simulink model "SimpleAdaptiveControl"  (R2017b)
settings: Solver=ode4  StartTime=0.0  StopTime=tsim  FixedStep=baseRate  RelTol=1e-3  EnableMultiTasking=on
values from neighbouring files (symbols this model uses):
  alpha = 1    [Run_Initializer.m]
  Cmout = [alpha*eye(3,3),eye(3,3)]    [Run_Initializer.m]
  drop_states_BLACK = [1.79313305664063,1.22521911621094,0.176047682762146]    [Run_Initializer.m]
  drop_states_RED = [2.60644311523438,1.21791186523438,3.08142089843750]    [Run_Initializer.m]
  GeI = 2e-2*eye(3,3)    [Run_Initializer.m]
  GeP = 1e-0*eye(3,3)    [Run_Initializer.m]
  GuI = 1e-2*eye(3,3)    [Run_Initializer.m]
  GuP = 8e-0*eye(3,3)    [Run_Initializer.m]
  GxI = 1e-2*eye(6,6)    [Run_Initializer.m]
  GxP = 8e-0*eye(6,6)    [Run_Initializer.m]
  home_states_BLACK = [ xLength/2; yLength/2; 0]    [Run_Initializer.m]
  home_states_RED = [ xLength/2+0.7; yLength/2; pi]    [Run_Initializer.m]
  init_states_BLACK = [ xLength/2; yLength/2; 0]    [Run_Initializer.m]
  init_states_RED = [ xLength/2+0.7; yLength/2; pi]    [Run_Initializer.m]
  Kd_tb = 0.4    [Run_Initializer.m]
  Kd_tr = 0.4    [Run_Initializer.m]
  Kd_xb = 5    [Run_Initializer.m]
  Kd_xr = 5    [Run_Initializer.m]
  Kd_yb = 5    [Run_Initializer.m]
  Kd_yr = 5    [Run_Initializer.m]
  KeI0 = (1e-4).*[   0.1063   -0.0058         0 ... (first row only)    [Run_Initializer.m]
  Kp_tb = 0.1    [Run_Initializer.m]
  Kp_tr = 0.1    [Run_Initializer.m]
  Kp_xb = 2    [Run_Initializer.m]
  Kp_xr = 2    [Run_Initializer.m]
  Kp_yb = 2    [Run_Initializer.m]
  Kp_yr = 2    [Run_Initializer.m]
  KuI0 = [  -0.0066   -0.0031         0 ... (first row only)    [Run_Initializer.m]
  KxI0 = [  -0.0060   -0.0020         0   -0.0001   -0.0001     0 ... (first row only)    [Run_Initializer.m]
  noise_variance_BLACK = 0    [Run_Initializer.m]
  noise_variance_RED = 0    [Run_Initializer.m]
  Phase0_End = Phase0_Duration    (= 10)    [Run_Initializer.m]
  Phase1_End = Phase0_Duration + Phase1_Duration    (= 15)    [Run_Initializer.m]
  Phase2_End = Phase0_Duration + Phase1_Duration +                                   Phase2_Duration    (= 35)    [Run_Initializer.m]
  Phase3_End = Phase0_Duration + Phase1_Duration +                                   Phase2_Duration + Phase3_Duration    (= 166)    [Run_Initializer.m]
  Phase3_SubPhase1_End = Phase2_End + Phase3_SubPhase1_Duration    (= 40)    [Run_Initializer.m]
  Phase3_SubPhase2_End = Phase2_End + Phase3_SubPhase1_Duration +                                   Phase3_SubPhase2_Duration    (= 45)    [Run_Initializer.m]
  Phase3_SubPhase3_End = Phase2_End + Phase3_SubPhase1_Duration +                                   Phase3_SubPhase2_Duration +                                  Phase3_SubPhase3_Duration    (= 46)    [Run_Initializer.m]
  Phase3_SubPhase4_End = Phase2_End + Phase3_SubPhase1_Duration +                                   Phase3_SubPhase2_Duration +                                  Phase3_SubPhase3_Duration +                                  Phase3_SubPhase4_Duration    [Run_Initializer.m]
  Phase4_End = Phase0_Duration + Phase1_Duration +                                   Phase2_Duration + Phase3_Duration +                                   Phase4_Duration    (= 186)    [Run_Initializer.m]
  Phase5_End = Phase0_Duration + Phase1_Duration +                                   Phase2_Duration + Phase3_Duration +                                   Phase4_Duration + Phase5_Duration    (= 191)    [Run_Initializer.m]
  serverRate = 0.1    [Run_Initializer.m]
  sigma_eI = 0.4    [Run_Initializer.m]
  sigma_uI = 0.4    [Run_Initializer.m]
  sigma_xI = 0.4    [Run_Initializer.m]
  sysd1 = c2d(sys,serverRate,opt)    [Run_Initializer.m]
  xLength = 3.51155    [Run_Initializer.m]
  xm_ini = [xLength/2+0.7, yLength/2, 0, 0, 0, 0]'    [Run_Initializer.m]
  yLength = 2.41935    [Run_Initializer.m]
undefined symbols (not defined in the file or in its folder): DiscIntNeverNeededParam, F_thrusters_BLACK, F_thrusters_RED, platformSelection, simMode, thruster_dist2CG_BLACK, thruster_dist2CG_RED
libraries: MainLibrary x22, GPIOLibrary x20, raspberrypilib x17, embdlinuxlib x6, dspsigops x5, dspswit3 x2
(part 1 of 5)
settings Model: Creator=AlexC  LastModifiedBy=SRCL
settings SolverCC: PositivePriorityOrder=on
settings OptimizationCC: UseFloatMulNetSlope=on  PassReuseOutputArgsThreshold=0  EfficientFloat2IntCast=on  MaxStackSize=64  SimCompilerOptimization=on
settings DebuggingCC: MultiTaskDSMMsg=none  ParameterTunabilityLossMsg=error
settings HardwareCC: ProdBitPerPointer=32  ProdBitPerSizeT=32  ProdBitPerPtrDiffT=32  ProdLargestAtomicInteger=Long  ProdLargestAtomicFloat=Double  ProdWordSize=32  ProdHWDeviceType=ARM Compatible->ARM Cortex
settings SFSimCC: MATLABDynamicMemAlloc=off
settings RTWCC: SystemTargetFile=ert.tlc  HardwareBoard=Raspberry Pi  TemplateMakefile=ert_default_tmf  Toolchain=GNU GCC Raspberry Pi  BuildConfiguration=Faster Runs  TargetLang=C++
settings CodeAppCC: ForceParamTrailComments=on  OperatorAnnotations=on
settings ERTTargetCC: TargetLangStandard=C++03 (ISO)  CombineSignalStateStructs=on  ERTCustomFileBanners=off  MatFileLogging=on  SupportContinuousTime=on  SupportNonInlinedSFcns=on  RemoveResetFunc=off  SupportVariableSizeSignals=on  ModelStepFunctionPrototypeControlCompliant=off  RootIOFormat=Structure reference

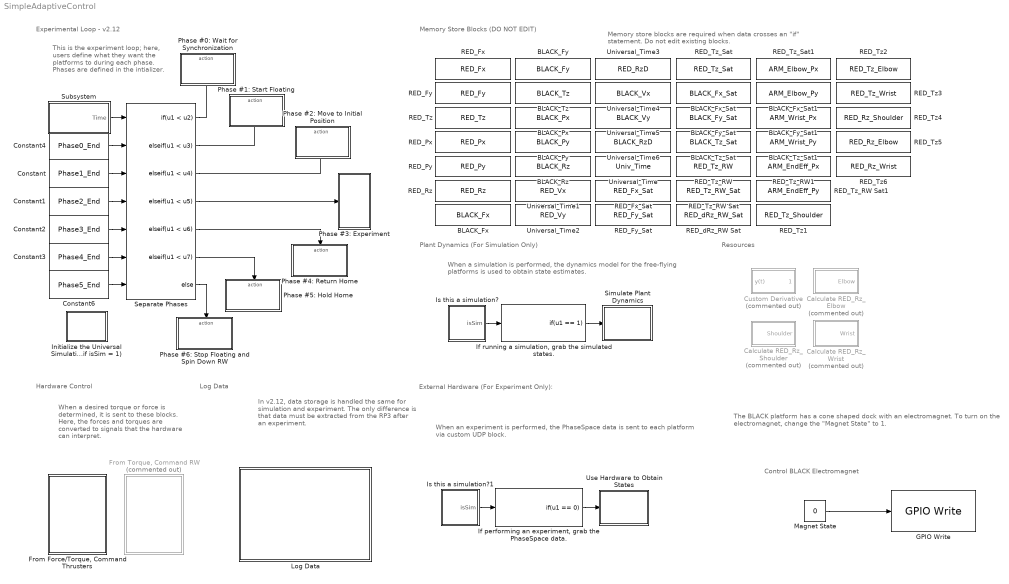
== system SimpleAdaptiveControl ==
  note: Hardware Control
  note: External Hardware (For Experiment Only):
  note: Experimental Loop - v2.12
  note: Log Data
  note: Memory Store Blocks (DO NOT EDIT)
  note: Plant Dynamics (For Simulation Only)
  note: This is the experiment loop; here, users define what they want the platforms to during each phase. Phases are defined in the intializer.
  note: When a desired torque or force is determined, it is sent to these blocks. Here, the forces and torques are converted to signals that the hardware can interpret.
  note: Memory store blocks are required when data crosses an "if" statement. Do not edit existing blocks.
  note: When a simulation is performed, the dynamics model for the free-flying platforms is used to obtain state estimates.
  note: When an experiment is performed, the PhaseSpace data is sent to each platform via custom UDP block.
  note: In v2.12, data storage is handled the same for simulation and experiment. The only difference is that data must be extracted from the RP3 after an experiment.
  note: Control BLACK Electromagnet
  note: The BLACK platform has a cone shaped dock with an electromagnet. To turn on the electromagnet, change the "Magnet State" to 1.
  note: Resources
  BLACK_Fx : DataStoreMemory  DataStoreName=BLACK_Fx  ReadBeforeWriteMsg=warning  WriteAfterWriteMsg=warning  WriteAfterReadMsg=warning  ShowAdditionalParam=off
  BLACK_Fx_Sat : DataStoreMemory  DataStoreName=BLACK_Fx_Sat  ReadBeforeWriteMsg=warning  WriteAfterWriteMsg=warning  WriteAfterReadMsg=warning  ShowAdditionalParam=off
  BLACK_Fx_Sat1 : DataStoreMemory  DataStoreName=ARM_Elbow_Py  ReadBeforeWriteMsg=warning  WriteAfterWriteMsg=warning  WriteAfterReadMsg=warning  ShowAdditionalParam=off
  BLACK_Fy : DataStoreMemory  DataStoreName=BLACK_Fy  ReadBeforeWriteMsg=warning  WriteAfterWriteMsg=warning  WriteAfterReadMsg=warning  ShowAdditionalParam=off
  BLACK_Fy_Sat : DataStoreMemory  DataStoreName=BLACK_Fy_Sat  ReadBeforeWriteMsg=warning  WriteAfterWriteMsg=warning  WriteAfterReadMsg=warning  ShowAdditionalParam=off
  BLACK_Fy_Sat1 : DataStoreMemory  DataStoreName=ARM_Wrist_Px  ReadBeforeWriteMsg=warning  WriteAfterWriteMsg=warning  WriteAfterReadMsg=warning  ShowAdditionalParam=off
  BLACK_Px : DataStoreMemory  DataStoreName=BLACK_Px  ReadBeforeWriteMsg=warning  WriteAfterWriteMsg=warning  WriteAfterReadMsg=warning  ShowAdditionalParam=off
  BLACK_Py : DataStoreMemory  DataStoreName=BLACK_Py  ReadBeforeWriteMsg=warning  WriteAfterWriteMsg=warning  WriteAfterReadMsg=warning  ShowAdditionalParam=off
  BLACK_Rz : DataStoreMemory  DataStoreName=BLACK_Rz  ReadBeforeWriteMsg=warning  WriteAfterWriteMsg=warning  WriteAfterReadMsg=warning  ShowAdditionalParam=off
  BLACK_Tz : DataStoreMemory  DataStoreName=BLACK_Tz  ReadBeforeWriteMsg=warning  WriteAfterWriteMsg=warning  WriteAfterReadMsg=warning  ShowAdditionalParam=off
  BLACK_Tz_Sat : DataStoreMemory  DataStoreName=BLACK_Tz_Sat  ReadBeforeWriteMsg=warning  WriteAfterWriteMsg=warning  WriteAfterReadMsg=warning  ShowAdditionalParam=off
  BLACK_Tz_Sat1 : DataStoreMemory  DataStoreName=ARM_Wrist_Py  ReadBeforeWriteMsg=warning  WriteAfterWriteMsg=warning  WriteAfterReadMsg=warning  ShowAdditionalParam=off
  Calculate RED_Rz_Elbow : Subsystem  Commented=on
  Calculate RED_Rz_Shoulder : Subsystem  Commented=on
  Calculate RED_Rz_Wrist : Subsystem  Commented=on
  Constant : Constant  Value=Phase1_End  SampleTime=-1
  Constant1 : Constant  Value=Phase2_End  SampleTime=-1
  Constant2 : Constant  Value=Phase3_End  SampleTime=-1
  Constant3 : Constant  Value=Phase4_End  SampleTime=-1
  Constant4 : Constant  Value=Phase0_End  SampleTime=-1
  Constant6 : Constant  Value=Phase5_End  SampleTime=-1
  Custom Derivative : Subsystem  Commented=on
  "From Force/Torque, Command Thrusters" : Subsystem  SystemSampleTime=0.1
  "From Torque, Command RW" : Subsystem  Commented=on
  GPIO Write : embdlinuxlib/GPIO Write  board=Pi 3 Model B  gpio=10  direction=Output  blockPlatform=Raspberry Pi
      settings: SourceProductName=Simulink Support Package for Raspberry Pi Hardware  SourceProductBaseCode=RASPPI
  "If performing an experiment, grab the PhaseSpace data." : If  IfExpression=u1 == 0  ShowElse=off
  "If running a simulation, grab the simulated states." : If  IfExpression=u1 == 1  ShowElse=off
  "Initialize the Universal Simulation Time (if isSim = 1) " : Subsystem
  Is this a simulation? : Subsystem
  Is this a simulation?1 : Subsystem
  Log Data : Subsystem
  Magnet State : Constant  Value=0
  Phase #0: Wait for Synchronization : Subsystem  TreatAsAtomicUnit=on
  "Phase #1: Start Floating " : Subsystem  TreatAsAtomicUnit=on
  Phase #2: Move to Initial Position : Subsystem  TreatAsAtomicUnit=on
  Phase #3: Experiment : Subsystem  TreatAsAtomicUnit=on
  Phase #4: Return Home : Subsystem  TreatAsAtomicUnit=on
  Phase #5: Hold Home : Subsystem  TreatAsAtomicUnit=on
  Phase #6: Stop Floating and Spin Down RW : Subsystem  TreatAsAtomicUnit=on
  RED_Fx : DataStoreMemory  DataStoreName=RED_Fx  ReadBeforeWriteMsg=warning  WriteAfterWriteMsg=warning  WriteAfterReadMsg=warning  ShowAdditionalParam=off
  RED_Fx_Sat : DataStoreMemory  DataStoreName=RED_Fx_Sat  ReadBeforeWriteMsg=warning  WriteAfterWriteMsg=warning  WriteAfterReadMsg=warning  ShowAdditionalParam=off
  RED_Fy : DataStoreMemory  DataStoreName=RED_Fy  ReadBeforeWriteMsg=warning  WriteAfterWriteMsg=warning  WriteAfterReadMsg=warning  ShowAdditionalParam=off
  RED_Fy_Sat : DataStoreMemory  DataStoreName=RED_Fy_Sat  ReadBeforeWriteMsg=warning  WriteAfterWriteMsg=warning  WriteAfterReadMsg=warning  ShowAdditionalParam=off
  RED_Px : DataStoreMemory  DataStoreName=RED_Px  ReadBeforeWriteMsg=warning  WriteAfterWriteMsg=warning  WriteAfterReadMsg=warning  ShowAdditionalParam=off
  RED_Py : DataStoreMemory  DataStoreName=RED_Py  ReadBeforeWriteMsg=warning  WriteAfterWriteMsg=warning  WriteAfterReadMsg=warning  ShowAdditionalParam=off
  RED_Rz : DataStoreMemory  DataStoreName=RED_Rz  ReadBeforeWriteMsg=warning  WriteAfterWriteMsg=warning  WriteAfterReadMsg=warning  ShowAdditionalParam=off
  RED_Tz : DataStoreMemory  DataStoreName=RED_Tz  ReadBeforeWriteMsg=warning  WriteAfterWriteMsg=warning  WriteAfterReadMsg=warning  ShowAdditionalParam=off
  RED_Tz1 : DataStoreMemory  DataStoreName=RED_Tz_Shoulder  ReadBeforeWriteMsg=warning  WriteAfterWriteMsg=warning  WriteAfterReadMsg=warning  ShowAdditionalParam=off
  RED_Tz2 : DataStoreMemory  DataStoreName=RED_Tz_Elbow  ReadBeforeWriteMsg=warning  WriteAfterWriteMsg=warning  WriteAfterReadMsg=warning  ShowAdditionalParam=off
  RED_Tz3 : DataStoreMemory  DataStoreName=RED_Tz_Wrist  ReadBeforeWriteMsg=warning  WriteAfterWriteMsg=warning  WriteAfterReadMsg=warning  ShowAdditionalParam=off
  RED_Tz4 : DataStoreMemory  DataStoreName=RED_Rz_Shoulder  ReadBeforeWriteMsg=warning  WriteAfterWriteMsg=warning  WriteAfterReadMsg=warning  ShowAdditionalParam=off
  RED_Tz5 : DataStoreMemory  DataStoreName=RED_Rz_Elbow  ReadBeforeWriteMsg=warning  WriteAfterWriteMsg=warning  WriteAfterReadMsg=warning  ShowAdditionalParam=off
  RED_Tz6 : DataStoreMemory  DataStoreName=RED_Rz_Wrist  ReadBeforeWriteMsg=warning  WriteAfterWriteMsg=warning  WriteAfterReadMsg=warning  ShowAdditionalParam=off
  RED_Tz_RW : DataStoreMemory  DataStoreName=RED_Tz_RW  ReadBeforeWriteMsg=warning  WriteAfterWriteMsg=warning  WriteAfterReadMsg=warning  ShowAdditionalParam=off
  RED_Tz_RW Sat : DataStoreMemory  DataStoreName=RED_Tz_RW_Sat  ReadBeforeWriteMsg=warning  WriteAfterWriteMsg=warning  WriteAfterReadMsg=warning  ShowAdditionalParam=off
  RED_Tz_RW Sat1 : DataStoreMemory  DataStoreName=ARM_EndEff_Py  ReadBeforeWriteMsg=warning  WriteAfterWriteMsg=warning  WriteAfterReadMsg=warning  ShowAdditionalParam=off
  RED_Tz_RW1 : DataStoreMemory  DataStoreName=ARM_EndEff_Px  ReadBeforeWriteMsg=warning  WriteAfterWriteMsg=warning  WriteAfterReadMsg=warning  ShowAdditionalParam=off
  RED_Tz_Sat : DataStoreMemory  DataStoreName=RED_Tz_Sat  ReadBeforeWriteMsg=warning  WriteAfterWriteMsg=warning  WriteAfterReadMsg=warning  ShowAdditionalParam=off
  RED_Tz_Sat1 : DataStoreMemory  DataStoreName=ARM_Elbow_Px  ReadBeforeWriteMsg=warning  WriteAfterWriteMsg=warning  WriteAfterReadMsg=warning  ShowAdditionalParam=off
  RED_dRz_RW Sat : DataStoreMemory  DataStoreName=RED_dRz_RW_Sat  ReadBeforeWriteMsg=warning  WriteAfterWriteMsg=warning  WriteAfterReadMsg=warning  ShowAdditionalParam=off
  Separate Phases : If  NumInputs=7  IfExpression=u1 < u2  ElseIfExpressions=u1 < u3, u1 < u4, u1 < u5, u1 < u6, u1 < u7
  Simulate Plant Dynamics : Subsystem  TreatAsAtomicUnit=on
  Subsystem : Subsystem
  Universal_Time : DataStoreMemory  DataStoreName=Univ_Time  ReadBeforeWriteMsg=warning  WriteAfterWriteMsg=warning  WriteAfterReadMsg=warning  ShowAdditionalParam=off
  Universal_Time1 : DataStoreMemory  DataStoreName=RED_Vx  ReadBeforeWriteMsg=warning  WriteAfterWriteMsg=warning  WriteAfterReadMsg=warning  ShowAdditionalParam=off
  Universal_Time2 : DataStoreMemory  DataStoreName=RED_Vy  ReadBeforeWriteMsg=warning  WriteAfterWriteMsg=warning  WriteAfterReadMsg=warning  ShowAdditionalParam=off
  Universal_Time3 : DataStoreMemory  DataStoreName=RED_RzD  ReadBeforeWriteMsg=warning  WriteAfterWriteMsg=warning  WriteAfterReadMsg=warning  ShowAdditionalParam=off
  Universal_Time4 : DataStoreMemory  DataStoreName=BLACK_Vx  ReadBeforeWriteMsg=warning  WriteAfterWriteMsg=warning  WriteAfterReadMsg=warning  ShowAdditionalParam=off
  Universal_Time5 : DataStoreMemory  DataStoreName=BLACK_Vy  ReadBeforeWriteMsg=warning  WriteAfterWriteMsg=warning  WriteAfterReadMsg=warning  ShowAdditionalParam=off
  Universal_Time6 : DataStoreMemory  DataStoreName=BLACK_RzD  ReadBeforeWriteMsg=warning  WriteAfterWriteMsg=warning  WriteAfterReadMsg=warning  ShowAdditionalParam=off
  Use Hardware to Obtain States : Subsystem  TreatAsAtomicUnit=on
  wires:
  Separate Phases/7 -> Phase #6: Stop Floating and Spin Down RW/Action
  Separate Phases/4 -> Phase #3: Experiment/Action
  Separate Phases/1 -> Phase #0: Wait for Synchronization/Action
  Is this a simulation?/1(isSim) -> "If running a simulation, grab the simulated states."/1
  Separate Phases/2 -> "Phase #1: Start Floating "/Action
  Separate Phases/5 -> Phase #4: Return Home/Action
  "If running a simulation, grab the simulated states."/1 -> Simulate Plant Dynamics/Action
  "If performing an experiment, grab the PhaseSpace data."/1 -> Use Hardware to Obtain States/Action
  Separate Phases/3 -> Phase #2: Move to Initial Position/Action
  Subsystem/1(Time) -> Separate Phases/1
  Is this a simulation?1/1(isSim) -> "If performing an experiment, grab the PhaseSpace data."/1
  Constant3/1 -> Separate Phases/6
  Constant2/1 -> Separate Phases/5
  Constant1/1 -> Separate Phases/4
  Constant/1 -> Separate Phases/3
  Constant4/1 -> Separate Phases/2
  Magnet State/1 -> GPIO Write/1
  Constant6/1 -> Separate Phases/7
  Separate Phases/6 -> Phase #5: Hold Home/Action

== system SimpleAdaptiveControl/Calculate RED_Rz_Elbow ==
  Subsystem2 : Subsystem
  Unwrap1 : dspsigops/Unwrap  tol=pi  InputProcessing=Columns as channels (frame based)  running=off
  Wrap2Pi1 : MATLAB Function  TreatAsAtomicUnit=on
  Elbow : Outport
  wires:
  Wrap2Pi1/1(angle_rad_wrapped) -> Elbow/1
  Unwrap1/1 -> Wrap2Pi1/1(angle_rad)
  Subsystem2/1(Out1) -> Unwrap1/1

== system SimpleAdaptiveControl/Calculate RED_Rz_Shoulder ==
  Subsystem1 : Subsystem
  Unwrap : dspsigops/Unwrap  tol=pi  InputProcessing=Columns as channels (frame based)  running=off
  Wrap2Pi : MATLAB Function  TreatAsAtomicUnit=on
  Shoulder : Outport
  wires:
  Wrap2Pi/1(angle_rad_wrapped) -> Shoulder/1
  Unwrap/1 -> Wrap2Pi/1(angle_rad)
  Subsystem1/1(Out1) -> Unwrap/1

== system SimpleAdaptiveControl/Calculate RED_Rz_Wrist ==
  Subsystem3 : Subsystem
  Unwrap2 : dspsigops/Unwrap  tol=pi  InputProcessing=Columns as channels (frame based)  running=off
  Wrap2Pi2 : MATLAB Function  TreatAsAtomicUnit=on
  Wrist : Outport
  wires:
  Wrap2Pi2/1(angle_rad_wrapped) -> Wrist/1
  Subsystem3/1(Out1) -> Unwrap2/1
  Unwrap2/1 -> Wrap2Pi2/1(angle_rad)

== system SimpleAdaptiveControl/Custom Derivative ==
  note: dy/dt ~= (y2-y1)/deltaT
  y(t) : Inport
  Delay1 : Delay  DelayLength=1  InitialConditionSource=Input port
      settings: InputPortMap=u0,p4
  Hold this value : Subsystem  TreatAsAtomicUnit=on
  Sum6 : Sum  Inputs=-+|
  divide by delta T : Gain  Gain=1/serverRate
  "if we went through a \"step\"" : If  IfExpression=u1 ~= 0  ShowElse=off
  dy(t)/dt : Outport
  wires:
  divide by delta T/1 -> dy(t)/dt/1
  Delay1/1 -> Sum6/1
  "if we went through a \"step\""/1 -> Hold this value/Action
  Hold this value/1(Out1) -> divide by delta T/1
  Sum6/1 -> "if we went through a \"step\""/1, Hold this value/1(In1)
  y(t)/1 -> Sum6/2, Delay1/2, Delay1/1

== system SimpleAdaptiveControl/From Force//Torque, Command Thrusters ==
  note: In this subsection, the "if" statements are used to determine two things: 1) whether or not a simulation is begin performed,
      | then 2) if an experiment is being performed, then which platform is the diagram compiled on. The "IdentifyPlatform" variable
      | is obtained from a text file location on each platform; each text file contains a unique identifier for each platform.
  note: To change the behavior of RED during this phase, double click on the "Change RED Behavior". For BLACK, double click on "Change BLACK Behavior"
  Change BLACK Behavior : Subsystem  TreatAsAtomicUnit=on
  Change RED Behavior : Subsystem  TreatAsAtomicUnit=on
  Is this a simulation? : Subsystem
  MATLAB System1 : MainLibrary/Auxiliary Functions/MATLAB System  SampleTime=-1
      settings: SourceProductName=SPOT Custom Library
  MATLAB System2 : MainLibrary/Auxiliary Functions/MATLAB System  SampleTime=-1
      settings: SourceProductName=SPOT Custom Library
  This IF block determines whether or not to run the BLACK sim/exp : If  NumInputs=2  IfExpression=u1 == 2 | u2 == 1  ShowElse=off
  "This IF block determines whether or not to run the RED sim/exp " : If  NumInputs=2  IfExpression=u1 == 1 | u2 == 1  ShowElse=off
  wires:
  Is this a simulation?/1(isSim) -> This IF block determines whether or not to run the BLACK sim/exp/2, "This IF block determines whether or not to run the RED sim/exp "/2
  "This IF block determines whether or not to run the RED sim/exp "/1 -> Change RED Behavior/Action
  This IF block determines whether or not to run the BLACK sim/exp/1 -> Change BLACK Behavior/Action
  MATLAB System1/1 -> "This IF block determines whether or not to run the RED sim/exp "/1
  MATLAB System2/1 -> This IF block determines whether or not to run the BLACK sim/exp/1

== system SimpleAdaptiveControl/From Torque, Command RW ==
  note: In this subsection, the "if" statements are used to determine two things: 1) whether or not a simulation is begin performed,
      | then 2) if an experiment is being performed, then which platform is the diagram compiled on. The "IdentifyPlatform" variable
      | is obtained from a text file location on each platform; each text file contains a unique identifier for each platform.
  note: To change the behavior of RED during this phase, double click on the "Change RED Behavior". For BLACK, double click on "Change BLACK Behavior"
  note: BUG HUNT: Last time the RW was tested, negative torques could not be applied.
  Change BLACK Behavior : Subsystem  TreatAsAtomicUnit=on
  Change RED Behavior : Subsystem  TreatAsAtomicUnit=on
  Is this a simulation? : Subsystem
  MATLAB System1 : MainLibrary/Auxiliary Functions/MATLAB System  SampleTime=-1
      settings: SourceProductName=SPOT Custom Library
  MATLAB System2 : MainLibrary/Auxiliary Functions/MATLAB System  SampleTime=-1
      settings: SourceProductName=SPOT Custom Library
  This IF block determines whether or not to run the BLACK sim/exp : If  NumInputs=2  IfExpression=u1 == 2 | u2 == 1  ShowElse=off
  "This IF block determines whether or not to run the RED sim/exp " : If  NumInputs=2  IfExpression=u1 == 1 | u2 == 1  ShowElse=off
  wires:
  Is this a simulation?/1(isSim) -> This IF block determines whether or not to run the BLACK sim/exp/2, "This IF block determines whether or not to run the RED sim/exp "/2
  "This IF block determines whether or not to run the RED sim/exp "/1 -> Change RED Behavior/Action
  This IF block determines whether or not to run the BLACK sim/exp/1 -> Change BLACK Behavior/Action
  MATLAB System1/1 -> "This IF block determines whether or not to run the RED sim/exp "/1
  MATLAB System2/1 -> This IF block determines whether or not to run the BLACK sim/exp/1

== system SimpleAdaptiveControl/Initialize the Universal Simulation Time (if isSim = 1)  ==
  note: When performing a simulation, the internal clock for the diagram is used instead of a universal time.
  "If this is a simulation, a clock must be initialized." : If  IfExpression=u1 == 1  ShowElse=off
  Initialize Universal Time (Simulation) : Subsystem  TreatAsAtomicUnit=on
  Is this a simulation? : Subsystem
  wires:
  Is this a simulation?/1(isSim) -> "If this is a simulation, a clock must be initialized."/1
  "If this is a simulation, a clock must be initialized."/1 -> Initialize Universal Time (Simulation)/Action

== system SimpleAdaptiveControl/Is this a simulation? ==
  Constant : Constant  Value=simMode  SampleTime=-1
  isSim : Outport
  wires:
  Constant/1 -> isSim/1

== system SimpleAdaptiveControl/Is this a simulation?1 ==
  Constant : Constant  Value=simMode  SampleTime=-1
  isSim : Outport
  wires:
  Constant/1 -> isSim/1

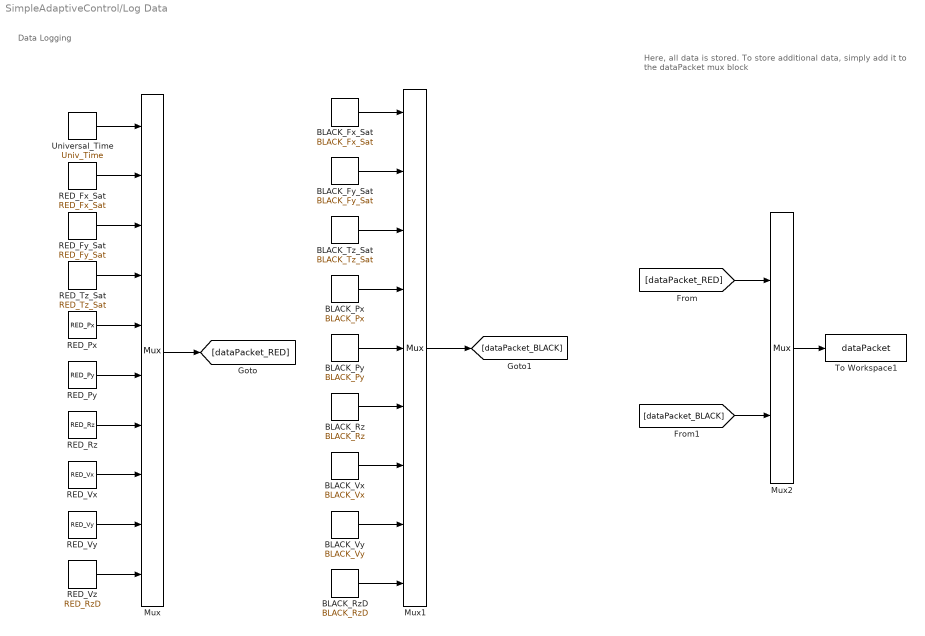
== system SimpleAdaptiveControl/Log Data ==
  note: Data Logging
  note: Here, all data is stored. To store additional data, simply add it to the dataPacket mux block
  BLACK_Fx_Sat : DataStoreRead  DataStoreName=BLACK_Fx_Sat
  BLACK_Fy_Sat : DataStoreRead  DataStoreName=BLACK_Fy_Sat
  BLACK_Px : DataStoreRead  DataStoreName=BLACK_Px
  BLACK_Py : DataStoreRead  DataStoreName=BLACK_Py
  BLACK_Rz : DataStoreRead  DataStoreName=BLACK_Rz
  BLACK_RzD : DataStoreRead  DataStoreName=BLACK_RzD
  BLACK_Tz_Sat : DataStoreRead  DataStoreName=BLACK_Tz_Sat
  BLACK_Vx : DataStoreRead  DataStoreName=BLACK_Vx
  BLACK_Vy : DataStoreRead  DataStoreName=BLACK_Vy
  Mux : Mux  Inputs=10
  Mux1 : Mux  Inputs=9
  Mux2 : Mux  Inputs=2
  RED_Fx_Sat : DataStoreRead  DataStoreName=RED_Fx_Sat
  RED_Fy_Sat : DataStoreRead  DataStoreName=RED_Fy_Sat
  RED_Px : DataStoreRead  DataStoreName=RED_Px
  "RED_Py " : DataStoreRead  DataStoreName=RED_Py
  RED_Rz : DataStoreRead  DataStoreName=RED_Rz
  RED_Tz_Sat : DataStoreRead  DataStoreName=RED_Tz_Sat
  "RED_Vx " : DataStoreRead  DataStoreName=RED_Vx
  RED_Vy : DataStoreRead  DataStoreName=RED_Vy
  RED_Vz : DataStoreRead  DataStoreName=RED_RzD
  To Workspace1 : ToWorkspace  VariableName=dataPacket  SampleTime=-1
      settings: Save2DSignal=2-D array (concatenate along first dimension)
  Universal_Time : DataStoreRead  DataStoreName=Univ_Time
  wires:
  "RED_Vx "/1 -> Mux/8
  RED_Vz/1 -> Mux/10
  RED_Px/1 -> Mux/5
  "RED_Py "/1 -> Mux/6
  RED_Vy/1 -> Mux/9
  RED_Fx_Sat/1 -> Mux/2
  RED_Rz/1 -> Mux/7
  RED_Fy_Sat/1 -> Mux/3
  RED_Tz_Sat/1 -> Mux/4
  Universal_Time/1 -> Mux/1
  BLACK_RzD/1 -> Mux1/9
  BLACK_Fx_Sat/1 -> Mux1/1
  BLACK_Fy_Sat/1 -> Mux1/2
  BLACK_Tz_Sat/1 -> Mux1/3
  BLACK_Vy/1 -> Mux1/8
  BLACK_Px/1 -> Mux1/4
  BLACK_Py/1 -> Mux1/5
  BLACK_Rz/1 -> Mux1/6
  BLACK_Vx/1 -> Mux1/7
  Mux/1 -> [dataPacket_RED]
  Mux1/1 -> [dataPacket_BLACK]
  [dataPacket_BLACK] -> Mux2/2
  [dataPacket_RED] -> Mux2/1
  Mux2/1 -> To Workspace1/1

== system SimpleAdaptiveControl/Phase #0: Wait for Synchronization ==
  note: In this subsection, the "if" statements are used to determine two things: 1) whether or not a simulation is begin performed,
      | then 2) if an experiment is being performed, then which platform is the diagram compiled on. The "IdentifyPlatform" variable
      | is obtained from a text file location on each platform; each text file contains a unique identifier for each platform.
  note: To change the behavior of RED during this phase, double click on the "Change RED Behavior". For BLACK, double click on "Change BLACK Behavior"
  Action Port : ActionPort  ActionType=then
  Change BLACK Behavior : Subsystem  TreatAsAtomicUnit=on
  Change RED Behavior : Subsystem  TreatAsAtomicUnit=on
  Is this a simulation? : Subsystem
  MATLAB System1 : MainLibrary/Auxiliary Functions/MATLAB System  SampleTime=-1
      settings: SourceProductName=SPOT Custom Library
  MATLAB System3 : MainLibrary/Auxiliary Functions/MATLAB System  SampleTime=-1
      settings: SourceProductName=SPOT Custom Library
  This IF block determines whether or not to run the BLACK sim/exp : If  NumInputs=2  IfExpression=u1 == 2 | u2 == 1  ShowElse=off
  "This IF block determines whether or not to run the RED sim/exp " : If  NumInputs=2  IfExpression=u1 == 1 | u2 == 1  ShowElse=off
  wires:
  MATLAB System3/1 -> "This IF block determines whether or not to run the RED sim/exp "/1
  Is this a simulation?/1(isSim) -> This IF block determines whether or not to run the BLACK sim/exp/2, "This IF block determines whether or not to run the RED sim/exp "/2
  "This IF block determines whether or not to run the RED sim/exp "/1 -> Change RED Behavior/Action
  This IF block determines whether or not to run the BLACK sim/exp/1 -> Change BLACK Behavior/Action
  MATLAB System1/1 -> This IF block determines whether or not to run the BLACK sim/exp/1

== system SimpleAdaptiveControl/Phase #1: Start Floating  ==
  note: In this subsection, the "if" statements are used to determine two things: 1) whether or not a simulation is begin performed,
      | then 2) if an experiment is being performed, then which platform is the diagram compiled on. The "IdentifyPlatform" variable
      | is obtained from a text file location on each platform; each text file contains a unique identifier for each platform.
  note: To change the behavior of RED during this phase, double click on the "Change RED Behavior". For BLACK, double click on "Change BLACK Behavior"
  Action Port : ActionPort  ActionType=elseif
  Change BLACK Behavior : Subsystem  TreatAsAtomicUnit=on
  Change RED Behavior : Subsystem  TreatAsAtomicUnit=on
  Is this a simulation? : Subsystem
  MATLAB System1 : MainLibrary/Auxiliary Functions/MATLAB System  SampleTime=-1
      settings: SourceProductName=SPOT Custom Library
  MATLAB System2 : MainLibrary/Auxiliary Functions/MATLAB System  SampleTime=-1
      settings: SourceProductName=SPOT Custom Library
  This IF block determines whether or not to run the BLACK sim/exp : If  NumInputs=2  IfExpression=u1 == 2 | u2 == 1  ShowElse=off
  "This IF block determines whether or not to run the RED sim/exp " : If  NumInputs=2  IfExpression=u1 == 1 | u2 == 1  ShowElse=off
  wires:
  MATLAB System1/1 -> "This IF block determines whether or not to run the RED sim/exp "/1
  "This IF block determines whether or not to run the RED sim/exp "/1 -> Change RED Behavior/Action
  Is this a simulation?/1(isSim) -> This IF block determines whether or not to run the BLACK sim/exp/2, "This IF block determines whether or not to run the RED sim/exp "/2
  MATLAB System2/1 -> This IF block determines whether or not to run the BLACK sim/exp/1
  This IF block determines whether or not to run the BLACK sim/exp/1 -> Change BLACK Behavior/Action

== system SimpleAdaptiveControl/Phase #2: Move to Initial Position ==
  note: In this subsection, the "if" statements are used to determine two things: 1) whether or not a simulation is begin performed,
      | then 2) if an experiment is being performed, then which platform is the diagram compiled on. The "IdentifyPlatform" variable
      | is obtained from a text file location on each platform; each text file contains a unique identifier for each platform.
  note: To change the behavior of RED during this phase, double click on the "Change RED Behavior". For BLACK, double click on "Change BLACK Behavior"
  Action Port : ActionPort  ActionType=elseif
  Change BLACK Behavior : Subsystem  TreatAsAtomicUnit=on
  Change RED Behavior : Subsystem  TreatAsAtomicUnit=on
  Is this a simulation? : Subsystem
  MATLAB System1 : MainLibrary/Auxiliary Functions/MATLAB System  SampleTime=-1
      settings: SourceProductName=SPOT Custom Library
  MATLAB System2 : MainLibrary/Auxiliary Functions/MATLAB System  SampleTime=-1
      settings: SourceProductName=SPOT Custom Library
  This IF block determines whether or not to run the BLACK sim/exp : If  NumInputs=2  IfExpression=u1 == 2 | u2 == 1  ShowElse=off
  "This IF block determines whether or not to run the RED sim/exp " : If  NumInputs=2  IfExpression=u1 == 1 | u2 == 1  ShowElse=off
  wires:
  MATLAB System2/1 -> This IF block determines whether or not to run the BLACK sim/exp/1
  This IF block determines whether or not to run the BLACK sim/exp/1 -> Change BLACK Behavior/Action
  Is this a simulation?/1(isSim) -> This IF block determines whether or not to run the BLACK sim/exp/2, "This IF block determines whether or not to run the RED sim/exp "/2
  "This IF block determines whether or not to run the RED sim/exp "/1 -> Change RED Behavior/Action
  MATLAB System1/1 -> "This IF block determines whether or not to run the RED sim/exp "/1

== system SimpleAdaptiveControl/Phase #3: Experiment ==
  note: To change the behavior of RED during this phase, double click on the "Change RED Behavior". For BLACK, double click on "Change BLACK Behavior"
  note: In this subsection, the "if" statements are used to determine two things: 1) whether or not a simulation is begin performed,
      | then 2) if an experiment is being performed, then which platform is the diagram compiled on. The "IdentifyPlatform" variable
      | is obtained from a text file location on each platform; each text file contains a unique identifier for each platform.
  Action Port : ActionPort  ActionType=elseif
  Change BLACK Behavior : Subsystem  TreatAsAtomicUnit=on
  Change RED Behavior : Subsystem  TreatAsAtomicUnit=on
  Is this a simulation? : Subsystem
  MATLAB System1 : MainLibrary/Auxiliary Functions/MATLAB System  SampleTime=-1
      settings: SourceProductName=SPOT Custom Library
  MATLAB System2 : MainLibrary/Auxiliary Functions/MATLAB System  SampleTime=-1
      settings: SourceProductName=SPOT Custom Library
  This IF block determines whether or not to run the BLACK sim/exp : If  NumInputs=2  IfExpression=u1 == 2 | u2 == 1  ShowElse=off
  "This IF block determines whether or not to run the RED sim/exp " : If  NumInputs=2  IfExpression=u1 == 1 | u2 == 1  ShowElse=off
  wires:
  MATLAB System2/1 -> This IF block determines whether or not to run the BLACK sim/exp/1
  "This IF block determines whether or not to run the RED sim/exp "/1 -> Change RED Behavior/Action
  Is this a simulation?/1(isSim) -> This IF block determines whether or not to run the BLACK sim/exp/2, "This IF block determines whether or not to run the RED sim/exp "/2
  MATLAB System1/1 -> "This IF block determines whether or not to run the RED sim/exp "/1
  This IF block determines whether or not to run the BLACK sim/exp/1 -> Change BLACK Behavior/Action

== system SimpleAdaptiveControl/Phase #4: Return Home ==
  note: In this subsection, the "if" statements are used to determine two things: 1) whether or not a simulation is begin performed,
      | then 2) if an experiment is being performed, then which platform is the diagram compiled on. The "IdentifyPlatform" variable
      | is obtained from a text file location on each platform; each text file contains a unique identifier for each platform.
  note: To change the behavior of RED during this phase, double click on the "Change RED Behavior". For BLACK, double click on "Change BLACK Behavior"
  Action Port : ActionPort  ActionType=elseif
  Change BLACK Behavior : Subsystem  TreatAsAtomicUnit=on
  Change RED Behavior : Subsystem  TreatAsAtomicUnit=on
  Is this a simulation? : Subsystem
  MATLAB System1 : MainLibrary/Auxiliary Functions/MATLAB System  SampleTime=-1
      settings: SourceProductName=SPOT Custom Library
  MATLAB System2 : MainLibrary/Auxiliary Functions/MATLAB System  SampleTime=-1
      settings: SourceProductName=SPOT Custom Library
  This IF block determines whether or not to run the BLACK sim/exp : If  NumInputs=2  IfExpression=u1 == 2 | u2 == 1  ShowElse=off
  "This IF block determines whether or not to run the RED sim/exp " : If  NumInputs=2  IfExpression=u1 == 1 | u2 == 1  ShowElse=off
  wires:
  MATLAB System2/1 -> This IF block determines whether or not to run the BLACK sim/exp/1
  "This IF block determines whether or not to run the RED sim/exp "/1 -> Change RED Behavior/Action
  Is this a simulation?/1(isSim) -> This IF block determines whether or not to run the BLACK sim/exp/2, "This IF block determines whether or not to run the RED sim/exp "/2
  MATLAB System1/1 -> "This IF block determines whether or not to run the RED sim/exp "/1
  This IF block determines whether or not to run the BLACK sim/exp/1 -> Change BLACK Behavior/Action

== system SimpleAdaptiveControl/Phase #5: Hold Home ==
  note: In this subsection, the "if" statements are used to determine two things: 1) whether or not a simulation is begin performed,
      | then 2) if an experiment is being performed, then which platform is the diagram compiled on. The "IdentifyPlatform" variable
      | is obtained from a text file location on each platform; each text file contains a unique identifier for each platform.
  note: To change the behavior of RED during this phase, double click on the "Change RED Behavior". For BLACK, double click on "Change BLACK Behavior"
  Action Port : ActionPort  ActionType=elseif
  Change BLACK Behavior : Subsystem  TreatAsAtomicUnit=on
  Change RED Behavior : Subsystem  TreatAsAtomicUnit=on
  Is this a simulation? : Subsystem
  MATLAB System1 : MainLibrary/Auxiliary Functions/MATLAB System  SampleTime=-1
      settings: SourceProductName=SPOT Custom Library
  MATLAB System2 : MainLibrary/Auxiliary Functions/MATLAB System  SampleTime=-1
      settings: SourceProductName=SPOT Custom Library
  This IF block determines whether or not to run the BLACK sim/exp : If  NumInputs=2  IfExpression=u1 == 2 | u2 == 1  ShowElse=off
  "This IF block determines whether or not to run the RED sim/exp " : If  NumInputs=2  IfExpression=u1 == 1 | u2 == 1  ShowElse=off
  wires:
  MATLAB System2/1 -> This IF block determines whether or not to run the BLACK sim/exp/1
  "This IF block determines whether or not to run the RED sim/exp "/1 -> Change RED Behavior/Action
  Is this a simulation?/1(isSim) -> This IF block determines whether or not to run the BLACK sim/exp/2, "This IF block determines whether or not to run the RED sim/exp "/2
  MATLAB System1/1 -> "This IF block determines whether or not to run the RED sim/exp "/1
  This IF block determines whether or not to run the BLACK sim/exp/1 -> Change BLACK Behavior/Action

== system SimpleAdaptiveControl/Phase #6: Stop Floating and Spin Down RW ==
  note: In this subsection, the "if" statements are used to determine two things: 1) whether or not a simulation is begin performed,
      | then 2) if an experiment is being performed, then which platform is the diagram compiled on. The "IdentifyPlatform" variable
      | is obtained from a text file location on each platform; each text file contains a unique identifier for each platform.
  note: To change the behavior of RED during this phase, double click on the "Change RED Behavior". For BLACK, double click on "Change BLACK Behavior"
  Action Port : ActionPort  ActionType=else
  Change BLACK Behavior : Subsystem  TreatAsAtomicUnit=on
  Change RED Behavior : Subsystem  TreatAsAtomicUnit=on
  Is this a simulation? : Subsystem
  MATLAB System1 : MainLibrary/Auxiliary Functions/MATLAB System  SampleTime=-1
      settings: SourceProductName=SPOT Custom Library
  MATLAB System2 : MainLibrary/Auxiliary Functions/MATLAB System  SampleTime=-1
      settings: SourceProductName=SPOT Custom Library
  This IF block determines whether or not to run the BLACK sim/exp : If  NumInputs=2  IfExpression=u1 == 2 | u2 == 1  ShowElse=off
  "This IF block determines whether or not to run the RED sim/exp " : If  NumInputs=2  IfExpression=u1 == 1 | u2 == 1  ShowElse=off
  wires:
  MATLAB System2/1 -> This IF block determines whether or not to run the BLACK sim/exp/1
  "This IF block determines whether or not to run the RED sim/exp "/1 -> Change RED Behavior/Action
  Is this a simulation?/1(isSim) -> This IF block determines whether or not to run the BLACK sim/exp/2, "This IF block determines whether or not to run the RED sim/exp "/2
  MATLAB System1/1 -> "This IF block determines whether or not to run the RED sim/exp "/1
  This IF block determines whether or not to run the BLACK sim/exp/1 -> Change BLACK Behavior/Action

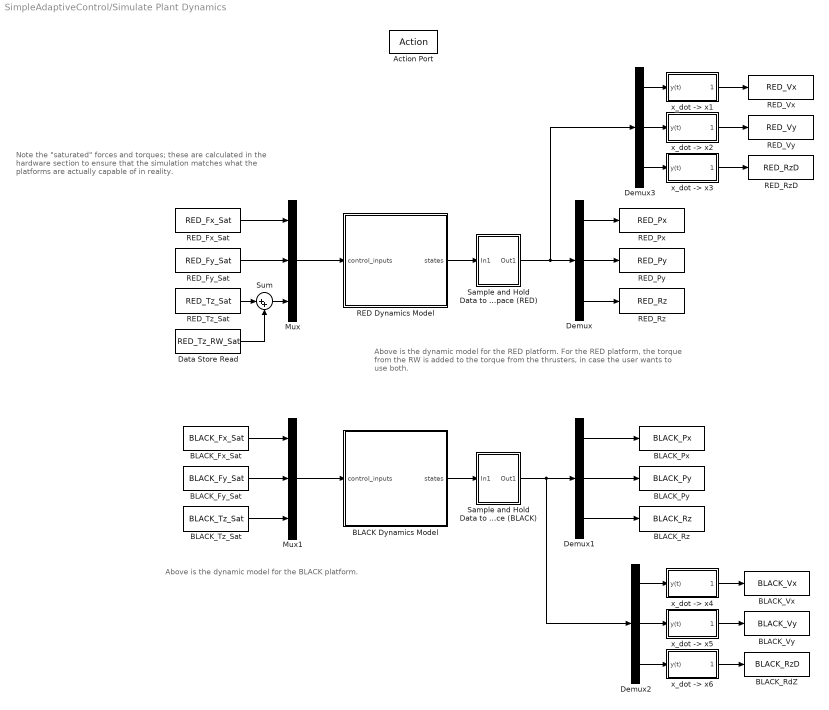
== system SimpleAdaptiveControl/Simulate Plant Dynamics ==
  note: Above is the dynamic model for the RED
      | platform. For the RED platform, the torque from the RW is added to the torque from the thrusters, in case the user wants to use both.
  note: Above is the dynamic model for the BLACK platform.
  note: Note the "saturated" forces and torques; these are calculated in the hardware section to ensure that the simulation matches what the platforms are actually capable of in reality.
  Action Port : ActionPort  ActionType=then
  BLACK Dynamics Model : Subsystem  SystemSampleTime=serverRate
  BLACK_Fx_Sat : DataStoreRead  DataStoreName=BLACK_Fx_Sat
  BLACK_Fy_Sat : DataStoreRead  DataStoreName=BLACK_Fy_Sat
  BLACK_Px : DataStoreWrite  DataStoreName=BLACK_Px
  BLACK_Py : DataStoreWrite  DataStoreName=BLACK_Py
  BLACK_RdZ : DataStoreWrite  DataStoreName=BLACK_RzD
  BLACK_Rz : DataStoreWrite  DataStoreName=BLACK_Rz
  BLACK_Tz_Sat : DataStoreRead  DataStoreName=BLACK_Tz_Sat
  BLACK_Vx : DataStoreWrite  DataStoreName=BLACK_Vx
  BLACK_Vy : DataStoreWrite  DataStoreName=BLACK_Vy
  Data Store Read : DataStoreRead  DataStoreName=RED_Tz_RW_Sat
  Demux{,1..3} (4 alike) : Demux  Outputs=3
  Mux : Mux  Inputs=3
  Mux1 : Mux  Inputs=3
  RED Dynamics Model : Subsystem  SystemSampleTime=serverRate
  RED_Fx_Sat : DataStoreRead  DataStoreName=RED_Fx_Sat
  RED_Fy_Sat : DataStoreRead  DataStoreName=RED_Fy_Sat
  RED_Px : DataStoreWrite  DataStoreName=RED_Px
  RED_Py : DataStoreWrite  DataStoreName=RED_Py
  RED_Rz : DataStoreWrite  DataStoreName=RED_Rz
  RED_RzD : DataStoreWrite  DataStoreName=RED_RzD
  RED_Tz_Sat : DataStoreRead  DataStoreName=RED_Tz_Sat
  RED_Vx : DataStoreWrite  DataStoreName=RED_Vx
  RED_Vy : DataStoreWrite  DataStoreName=RED_Vy
  Sample and Hold Data to Match PhaseSpace (BLACK) : Subsystem
  Sample and Hold Data to Match PhaseSpace (RED) : Subsystem
  Sum : Sum  Inputs=|++
  "x_dot -> x1" : Subsystem
  "x_dot -> x2" : Subsystem
  "x_dot -> x3" : Subsystem
  "x_dot -> x4" : Subsystem
  "x_dot -> x5" : Subsystem
  "x_dot -> x6" : Subsystem
  wires:
  Demux/3 -> RED_Rz/1
  RED_Fx_Sat/1 -> Mux/1
  BLACK_Fy_Sat/1 -> Mux1/2
  BLACK_Tz_Sat/1 -> Mux1/3
  RED_Fy_Sat/1 -> Mux/2
  BLACK_Fx_Sat/1 -> Mux1/1
  Demux/2 -> RED_Py/1
  Demux/1 -> RED_Px/1
  Demux1/1 -> BLACK_Px/1
  Demux1/2 -> BLACK_Py/1
  Demux1/3 -> BLACK_Rz/1
  RED_Tz_Sat/1 -> Sum/1
  Sum/1 -> Mux/3
  Data Store Read/1 -> Sum/2
  Demux2/1 -> "x_dot -> x4"/1(y(t))
  Demux2/2 -> "x_dot -> x5"/1(y(t))
  Demux2/3 -> "x_dot -> x6"/1(y(t))
  Demux3/2 -> "x_dot -> x2"/1(y(t))
  Demux3/1 -> "x_dot -> x1"/1(y(t))
  Demux3/3 -> "x_dot -> x3"/1(y(t))
  "x_dot -> x1"/1(dy(t)/dt) -> RED_Vx/1
  "x_dot -> x2"/1(dy(t)/dt) -> RED_Vy/1
  "x_dot -> x3"/1(dy(t)/dt) -> RED_RzD/1
  "x_dot -> x4"/1(dy(t)/dt) -> BLACK_Vx/1
  "x_dot -> x5"/1(dy(t)/dt) -> BLACK_Vy/1
  "x_dot -> x6"/1(dy(t)/dt) -> BLACK_RdZ/1
  Mux/1 -> RED Dynamics Model/1(control_inputs)
  Mux1/1 -> BLACK Dynamics Model/1(control_inputs)
  Sample and Hold Data to Match PhaseSpace (BLACK)/1(Out1) -> Demux2/1, Demux1/1
  BLACK Dynamics Model/1(states) -> Sample and Hold Data to Match PhaseSpace (BLACK)/1(In1)
  Sample and Hold Data to Match PhaseSpace (RED)/1(Out1) -> Demux3/1, Demux/1
  RED Dynamics Model/1(states) -> Sample and Hold Data to Match PhaseSpace (RED)/1(In1)

== system SimpleAdaptiveControl/Subsystem ==
  Universal_Time : DataStoreRead  DataStoreName=Univ_Time
  Time : Outport
  wires:
  Universal_Time/1 -> Time/1

== system SimpleAdaptiveControl/Use Hardware to Obtain States ==
  note: Because the UDP block binds to the first platofrm that it sees, it is not currently possible to run RED+BLACK without having RED send BLACK the data packets.
  Action Port : ActionPort  ActionType=then
  "Check whether both platforms are being used, and if so then use RED to send data to BLACK " : If  IfExpression=u1 == 1 | u1 == 2 | u1 == 5  ElseIfExpressions=u1 == 3| u1 == 4  ShowElse=off
  "Using RED+BLACK, or RED+BLACK+ARM" : Subsystem  TreatAsAtomicUnit=on
  "Using RED, BLACK, or RED + ARM" : Subsystem  TreatAsAtomicUnit=on
  Which PLATFORM is being used? : Constant  Value=platformSelection
  wires:
  "Check whether both platforms are being used, and if so then use RED to send data to BLACK "/1 -> "Using RED, BLACK, or RED + ARM"/Action
  Which PLATFORM is being used?/1 -> "Check whether both platforms are being used, and if so then use RED to send data to BLACK "/1
  "Check whether both platforms are being used, and if so then use RED to send data to BLACK "/2 -> "Using RED+BLACK, or RED+BLACK+ARM"/Action

== system SimpleAdaptiveControl/Calculate RED_Rz_Elbow/Subsystem2 ==
  Atan2 : Trigonometry  Operator=atan2
  Constant2 : Constant  Value=pi/2
  Data Store Read : DataStoreRead  DataStoreName=ARM_Wrist_Py
  Data Store Read1 : DataStoreRead  DataStoreName=ARM_Elbow_Py
  Data Store Read2 : DataStoreRead  DataStoreName=ARM_Wrist_Px
  Data Store Read3 : DataStoreRead  DataStoreName=ARM_Elbow_Px
  Data Store Read4 : DataStoreRead  DataStoreName=RED_Rz_Shoulder
  Data Store Read6 : DataStoreRead  DataStoreName=RED_Rz
  Subtract : Sum  Inputs=+-
  Subtract1 : Sum  Inputs=+-
  Subtract2 : Sum  Inputs=+---
  Out1 : Outport
  wires:
  Data Store Read1/1 -> Subtract/2
  Subtract/1 -> Atan2/1
  Data Store Read4/1 -> Subtract2/4
  Data Store Read/1 -> Subtract/1
  Data Store Read2/1 -> Subtract1/1
  Data Store Read3/1 -> Subtract1/2
  Subtract2/1 -> Out1/1
  Subtract1/1 -> Atan2/2
  Constant2/1 -> Subtract2/2
  Data Store Read6/1 -> Subtract2/3
  Atan2/1 -> Subtract2/1

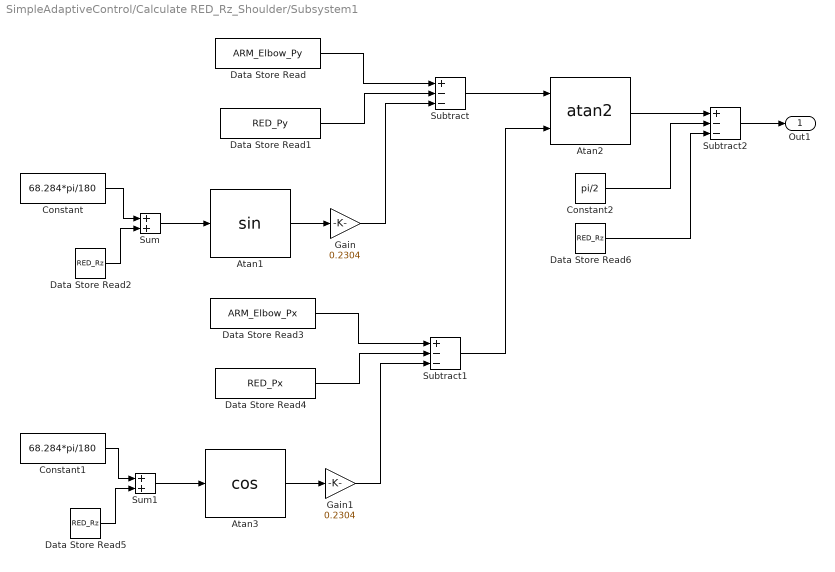
== system SimpleAdaptiveControl/Calculate RED_Rz_Shoulder/Subsystem1 ==
  Atan1 : Trigonometry
  Atan2 : Trigonometry  Operator=atan2
  Atan3 : Trigonometry  Operator=cos
  Constant : Constant  Value=68.284*pi/180
  Constant1 : Constant  Value=68.284*pi/180
  Constant2 : Constant  Value=pi/2
  Data Store Read : DataStoreRead  DataStoreName=ARM_Elbow_Py
  Data Store Read1 : DataStoreRead  DataStoreName=RED_Py
  Data Store Read2 : DataStoreRead  DataStoreName=RED_Rz
  Data Store Read3 : DataStoreRead  DataStoreName=ARM_Elbow_Px
  Data Store Read4 : DataStoreRead  DataStoreName=RED_Px
  Data Store Read5 : DataStoreRead  DataStoreName=RED_Rz
  Data Store Read6 : DataStoreRead  DataStoreName=RED_Rz
  Gain : Gain  Gain=0.2304
  Gain1 : Gain  Gain=0.2304
  Subtract : Sum  Inputs=+--
  Subtract1 : Sum  Inputs=+--
  Subtract2 : Sum  Inputs=+--
  Sum : Sum
  Sum1 : Sum
  Out1 : Outport
  wires:
  Data Store Read2/1 -> Sum/2
  Constant/1 -> Sum/1
  Constant1/1 -> Sum1/1
  Sum1/1 -> Atan3/1
  Atan3/1 -> Gain1/1
  Data Store Read4/1 -> Subtract1/2
  Data Store Read5/1 -> Sum1/2
  Data Store Read3/1 -> Subtract1/1
  Gain1/1 -> Subtract1/3
  Constant2/1 -> Subtract2/2
  Data Store Read/1 -> Subtract/1
  Atan2/1 -> Subtract2/1
  Subtract2/1 -> Out1/1
  Data Store Read6/1 -> Subtract2/3
  Data Store Read1/1 -> Subtract/2
  Subtract1/1 -> Atan2/2
  Gain/1 -> Subtract/3
  Sum/1 -> Atan1/1
  Atan1/1 -> Gain/1
  Subtract/1 -> Atan2/1

== system SimpleAdaptiveControl/Calculate RED_Rz_Wrist/Subsystem3 ==
  Atan2 : Trigonometry  Operator=atan2
  Constant2 : Constant  Value=pi/2
  Data Store Read : DataStoreRead  DataStoreName=ARM_Wrist_Py
  Data Store Read1 : DataStoreRead  DataStoreName=ARM_EndEff_Py
  Data Store Read2 : DataStoreRead  DataStoreName=ARM_Wrist_Px
  Data Store Read3 : DataStoreRead  DataStoreName=RED_Rz_Elbow
  Data Store Read4 : DataStoreRead  DataStoreName=RED_Rz_Shoulder
  Data Store Read5 : DataStoreRead  DataStoreName=ARM_EndEff_Px
  Data Store Read6 : DataStoreRead  DataStoreName=RED_Rz
  Subtract : Sum  Inputs=+-
  Subtract1 : Sum  Inputs=+-
  Subtract2 : Sum  Inputs=+----
  Out1 : Outport
  wires:
  Subtract/1 -> Atan2/1
  Data Store Read4/1 -> Subtract2/4
  Data Store Read2/1 -> Subtract1/2
  Subtract2/1 -> Out1/1
  Subtract1/1 -> Atan2/2
  Constant2/1 -> Subtract2/2
  Data Store Read6/1 -> Subtract2/3
  Atan2/1 -> Subtract2/1
  Data Store Read/1 -> Subtract/2
  Data Store Read1/1 -> Subtract/1
  Data Store Read5/1 -> Subtract1/1
  Data Store Read3/1 -> Subtract2/5

== system SimpleAdaptiveControl/Custom Derivative/Hold this value ==
  In1 : Inport
  Action Port : ActionPort
  Out1 : Outport
  wires:
  In1/1 -> Out1/1

== system SimpleAdaptiveControl/From Force//Torque, Command Thrusters/Change BLACK Behavior ==
  note: Calculate the percentage of time each thruster must be on, and send to the PWM blocks.
  note: For user reference, the Raspberry Pi 3 GPIO labels are shown below:
  note: Using the attitude, rotate the forces into the body frame.
  note: Calculate which thrusters must be turned on and for how long.
  Action Port : ActionPort  ActionType=then
  BLACK_Fx : DataStoreRead  DataStoreName=BLACK_Fx
  BLACK_Fy : DataStoreRead  DataStoreName=BLACK_Fy
  BLACK_Rz : DataStoreRead  DataStoreName=BLACK_Rz
  Calculate Thruster ON/OFF : Subsystem
  Mux : Mux  Inputs=2
  Mux1 : Mux  Inputs=2
  RED_Tz : DataStoreRead  DataStoreName=BLACK_Tz
  Rotate Forces to Body : Subsystem
  Subsystem : Subsystem  TreatAsAtomicUnit=on  SystemSampleTime=0.1
  wires:
  Rotate Forces to Body/1(F_b) -> Mux1/1
  BLACK_Fx/1 -> Mux/1
  Calculate Thruster ON/OFF/1(ThrusterPWM) -> Subsystem/1(Thruster PWM)
  BLACK_Rz/1 -> Rotate Forces to Body/2(Rz)
  Mux/1 -> Rotate Forces to Body/1("F_I ")
  RED_Tz/1 -> Mux1/2
  Mux1/1 -> Calculate Thruster ON/OFF/1("[Fx_b; Fy_b; Tz]")
  BLACK_Fy/1 -> Mux/2

== system SimpleAdaptiveControl/From Force//Torque, Command Thrusters/Change RED Behavior ==
  note: Calculate which thrusters must be turned on and for how long.
  note: Using the attitude, rotate the forces into the body frame.
  note: Calculate the percentage of time each thruster must be on, and send to the PWM blocks.
  Action Port : ActionPort  ActionType=then
  Calculate Thruster ON/OFF : Subsystem
  Mux : Mux  Inputs=2
  Mux1 : Mux  Inputs=2
  RED_Fx : DataStoreRead  DataStoreName=RED_Fx
  RED_Fy : DataStoreRead  DataStoreName=RED_Fy
  RED_Rz : DataStoreRead  DataStoreName=RED_Rz
  RED_Tz : DataStoreRead  DataStoreName=RED_Tz
  Rotate Forces to Body : Subsystem
  Subsystem : Subsystem  TreatAsAtomicUnit=on  SystemSampleTime=0.1
  wires:
  RED_Tz/1 -> Mux1/2
  Mux/1 -> Rotate Forces to Body/1("F_I ")
  RED_Fy/1 -> Mux/2
  Mux1/1 -> Calculate Thruster ON/OFF/1("[Fx_b; Fy_b; Tz]")
  RED_Fx/1 -> Mux/1
  RED_Rz/1 -> Rotate Forces to Body/2(Rz)
  Rotate Forces to Body/1(F_b) -> Mux1/1
  Calculate Thruster ON/OFF/1(ThrusterPWM) -> Subsystem/1(Thruster PWM)

== system SimpleAdaptiveControl/From Force//Torque, Command Thrusters/Is this a simulation? ==
  Constant : Constant  Value=simMode  SampleTime=-1
  isSim : Outport
  wires:
  Constant/1 -> isSim/1

== system SimpleAdaptiveControl/From Torque, Command RW/Change BLACK Behavior ==
  note: BLACK does not currently have the capability to use a RW.
  Action Port : ActionPort  ActionType=then

== system SimpleAdaptiveControl/From Torque, Command RW/Change RED Behavior ==
  note: In this subsection, the commanded torque is converted to an RPM, which is then saturated based on the known limits of the RW
  note: The saturated wheel RPM is then sent to the wheel controller using PWM blocks.
  Action Port : ActionPort  ActionType=then
  Calculate Saturated RPM Signal : Subsystem
  RED_Tz_RW : DataStoreRead  DataStoreName=RED_Tz_RW
  RED_Tz_RW_Sat : DataStoreWrite  DataStoreName=RED_Tz_RW_Sat
  Wheel RPM to PWM : Subsystem
  wires:
  Calculate Saturated RPM Signal/2(RPM_Sat) -> RED_Tz_RW_Sat/1
  RED_Tz_RW/1 -> Calculate Saturated RPM Signal/1(Tz)
  Calculate Saturated RPM Signal/1(RPM) -> Wheel RPM to PWM/1(WheelRPM)

== system SimpleAdaptiveControl/From Torque, Command RW/Is this a simulation? ==
  Constant : Constant  Value=simMode  SampleTime=-1
  isSim : Outport
  wires:
  Constant/1 -> isSim/1
